simulink model "Steering_dynamics_discrete_mdl"  (R2026a)
settings: Solver=VariableStepAuto  StopTime=1
undefined symbols (not defined in the file): Vehicle
(part 2 of 2)

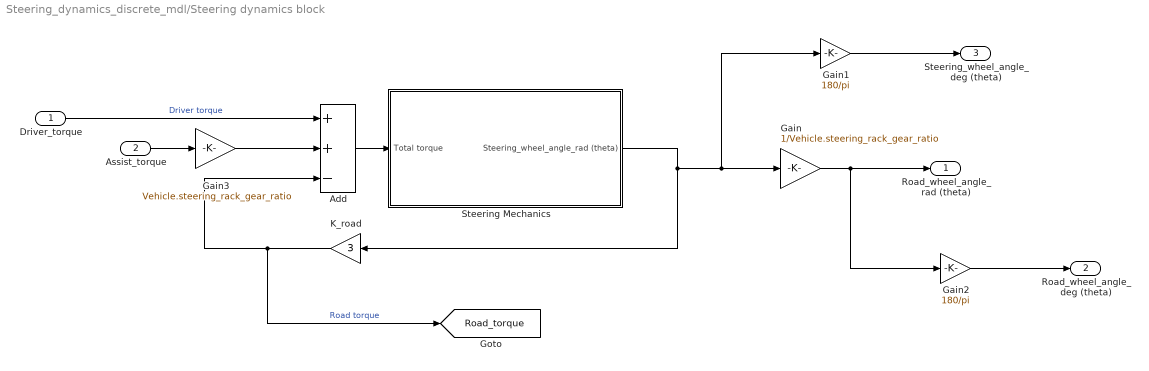
== system Steering_dynamics_discrete_mdl/Steering dynamics block ==
  Driver_torque : Inport
  Assist_torque : Inport  Port=2
  Add : Sum  Inputs=++-
  Gain : Gain  Gain=1/Vehicle.steering_rack_gear_ratio
  Gain1 : Gain  Gain=180/pi
  Gain2 : Gain  Gain=180/pi
  Gain3 : Gain  Gain=Vehicle.steering_rack_gear_ratio
  K_road : Gain  Gain=3
  Steering Mechanics : Subsystem
  Road_wheel_angle_rad (theta) : Outport
  Road_wheel_angle_deg (theta) : Outport  Port=2
  Steering_wheel_angle_deg (theta) : Outport  Port=3
  tag scope: Road_torque=global
  wires:
  Add/1 -> Steering Mechanics/1(Total torque)
  Steering Mechanics/1(Steering_wheel_angle_rad (theta)) -> Gain/1, Gain1/1, K_road/1
  K_road/1 -> [Road_torque], Add/3  "Road torque"
  Driver_torque/1 -> Add/1  "Driver torque"
  Gain/1 -> Road_wheel_angle_rad (theta)/1, Gain2/1
  Assist_torque/1 -> Gain3/1
  Gain1/1 -> Steering_wheel_angle_deg (theta)/1
  Gain2/1 -> Road_wheel_angle_deg (theta)/1
  Gain3/1 -> Add/2

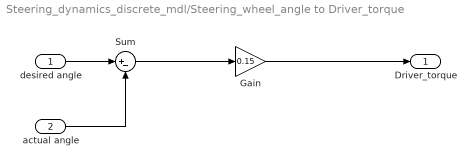
== system Steering_dynamics_discrete_mdl/Steering_wheel_angle to Driver_torque ==
  desired angle : Inport
  actual angle : Inport  Port=2
  Gain : Gain  Gain=0.15
  Sum : Sum  Inputs=|+-
  Driver_torque : Outport
  wires:
  desired angle/1 -> Sum/1
  actual angle/1 -> Sum/2
  Sum/1 -> Gain/1
  Gain/1 -> Driver_torque/1

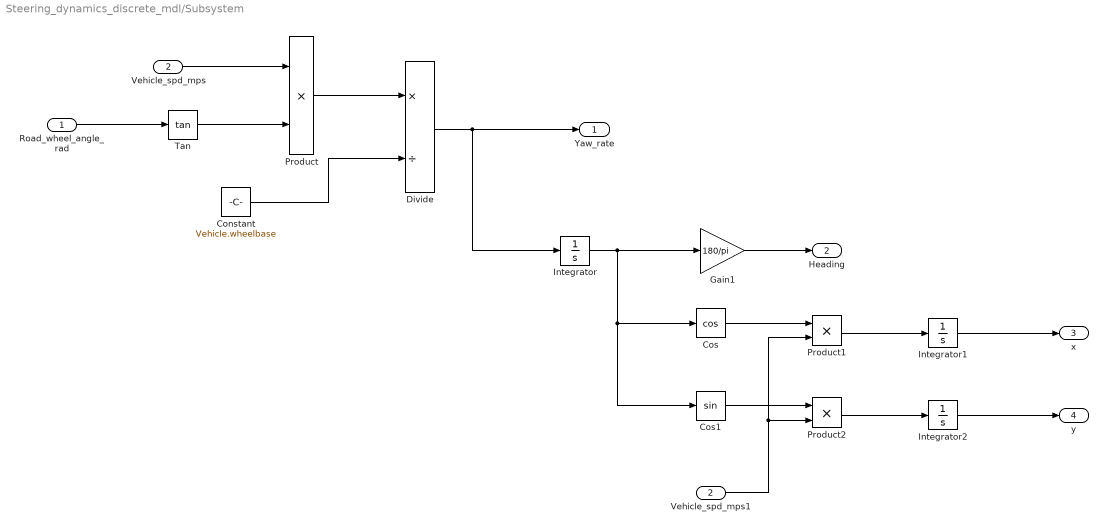
== system Steering_dynamics_discrete_mdl/Subsystem ==
  Road_wheel_angle_rad : Inport
  Vehicle_spd_mps : Inport  Port=2
  Constant : Constant  Value=Vehicle.wheelbase
  Cos : Trigonometry  Operator=cos
  Cos1 : Trigonometry
  Divide : Product  Inputs=*/
  Gain1 : Gain  Gain=180/pi
  Integrator : Integrator
  Integrator1 : Integrator
  Integrator2 : Integrator
  Product : Product
  Product1 : Product
  Product2 : Product
  Tan : Trigonometry  Operator=tan
  Vehicle_spd_mps1 : InportShadow  Port=2
  Yaw_rate : Outport
  Heading : Outport  Port=2
  x : Outport  Port=3
  y : Outport  Port=4
  wires:
  Road_wheel_angle_rad/1 -> Tan/1
  Tan/1 -> Product/2
  Vehicle_spd_mps/1 -> Product/1
  Product/1 -> Divide/1
  Constant/1 -> Divide/2
  Divide/1 -> Integrator/1, Yaw_rate/1
  Integrator/1 -> Cos/1, Cos1/1, Gain1/1
  Cos/1 -> Product1/1
  Vehicle_spd_mps1/1 -> Product2/2, Product1/2
  Cos1/1 -> Product2/1
  Product1/1 -> Integrator1/1
  Product2/1 -> Integrator2/1
  Integrator1/1 -> x/1
  Integrator2/1 -> y/1
  Gain1/1 -> Heading/1

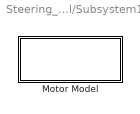
== system Steering_dynamics_discrete_mdl/Subsystem1 ==
  Motor Model : Subsystem

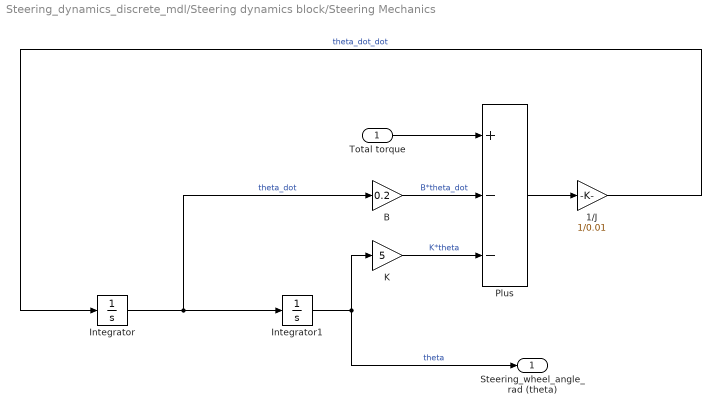
== system Steering_dynamics_discrete_mdl/Steering dynamics block/Steering Mechanics ==
  Total torque : Inport
  1/J : Gain  Gain=1/0.01
  B : Gain  Gain=0.2
  Integrator : Integrator
  Integrator1 : Integrator
  K : Gain  Gain=5
  Plus : Sum  Inputs=+--
  Steering_wheel_angle_rad (theta) : Outport
  wires:
  1/J/1 -> Integrator/1  "theta_dot_dot"
  Integrator/1 -> B/1, Integrator1/1  "theta_dot"
  Integrator1/1 -> Steering_wheel_angle_rad (theta)/1, K/1  "theta"
  B/1 -> Plus/2  "B*theta_dot"
  K/1 -> Plus/3  "K*theta"
  Plus/1 -> 1/J/1
  Total torque/1 -> Plus/1

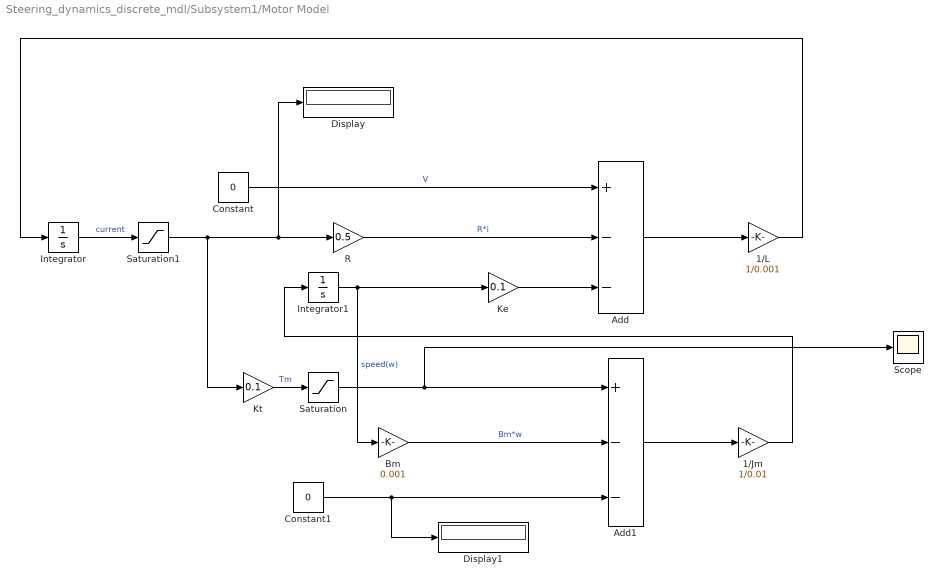
== system Steering_dynamics_discrete_mdl/Subsystem1/Motor Model ==
  1/Jm : Gain  Gain=1/0.01
  1/L : Gain  Gain=1/0.001
  Add : Sum  Inputs=+--
  Add1 : Sum  Inputs=+--
  Bm : Gain  Gain=0.001
  Constant : Constant  Value=0
  Constant1 : Constant  Value=0
  Display : Display
  Display1 : Display
  Integrator : Integrator
  Integrator1 : Integrator
  Ke : Gain  Gain=0.1
  Kt : Gain  Gain=0.1
  R : Gain  Gain=0.5
  Saturation : Saturate  UpperLimit=2  LowerLimit=-2
  Saturation1 : Saturate  UpperLimit=20  LowerLimit=-20
  Scope : Scope
      settings: ActiveDisplayYMinimum=-1  ActiveDisplayYMaximum=1  DataLoggingVariableName=ScopeData8
  wires:
  Constant/1 -> Add/1  "V"
  Integrator/1 -> Saturation1/1  "current"
  R/1 -> Add/2  "R*i"
  Integrator1/1 -> Ke/1, Bm/1  "speed(w)"
  Ke/1 -> Add/3
  Add/1 -> 1/L/1
  1/L/1 -> Integrator/1
  Kt/1 -> Saturation/1  "Tm"
  Bm/1 -> Add1/2  "Bm*w"
  Add1/1 -> 1/Jm/1
  1/Jm/1 -> Integrator1/1
  Constant1/1 -> Display1/1, Add1/3
  Saturation/1 -> Scope/1, Add1/1
  Saturation1/1 -> Kt/1, Display/1, R/1
